simulink model "PMSM"  (R2024b)
settings: Solver=VariableStepAuto  StartTime=0.0  StopTime=1  RelTol=1e-3
InitFcn:
  | Rs=2.98;
  | Ld=7*10^-3;
  | Lq=7*10^-3;
  | pm=0.125;
  | p=2;
  | B=11*10^-5;
  | J=0.47*10^-4;
libraries: spsPLL3phLib x1, spsabctoAlphaBetaZeroLib x1, spsabctodq0Lib x1
settings Model: Creator=krishanchoudhary  LastModifiedBy=krishanchoudhary

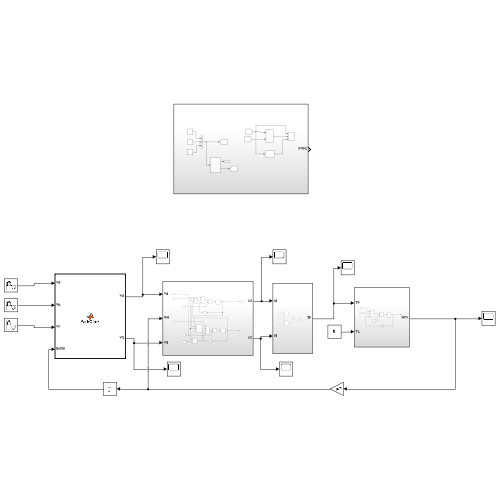
[thumbnail: Simulink's stored preview of the top-level diagram]
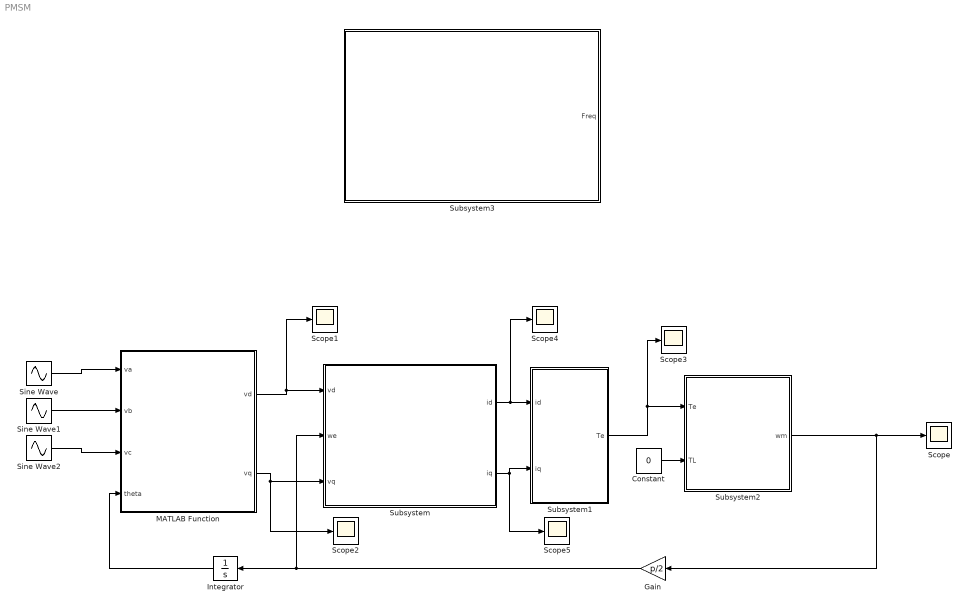
== system PMSM ==
  Constant : Constant  Value=0
  Gain : Gain  Gain=p/2
  Integrator : Integrator
  MATLAB Function : MATLAB Function  TreatAsAtomicUnit=on
  Scope{,1..5} (6 alike) : Scope
  Sine Wave : Sin  Amplitude=240  Frequency=2*pi*50  SampleTime=0.001
  Sine Wave1 : Sin  Amplitude=240  Frequency=2*pi*50  Phase=-(2*pi)/3  SampleTime=0.001
  Sine Wave2 : Sin  Amplitude=240  Frequency=2*pi*50  Phase=(2*pi)/3  SampleTime=0.001
  Subsystem : Subsystem
  Subsystem1 : Subsystem
  Subsystem2 : Subsystem
  Subsystem3 : Subsystem
  wires:
  Subsystem/1(id) -> Scope4/1, Subsystem1/1(id)
  Subsystem/2(iq) -> Scope5/1, Subsystem1/2(iq)
  Subsystem1/1(Te) -> Scope3/1, Subsystem2/1(Te)
  Constant/1 -> Subsystem2/2(TL)
  Subsystem2/1(wm) -> Scope/1, Gain/1
  MATLAB Function/1(vd) -> Scope1/1, Subsystem/1(vd)
  MATLAB Function/2(vq) -> Scope2/1, Subsystem/3(vq)
  Integrator/1 -> MATLAB Function/4(theta)
  Gain/1 -> Subsystem/2(we), Integrator/1
  Sine Wave/1 -> MATLAB Function/1(va)
  Sine Wave1/1 -> MATLAB Function/2(vb)
  Sine Wave2/1 -> MATLAB Function/3(vc)

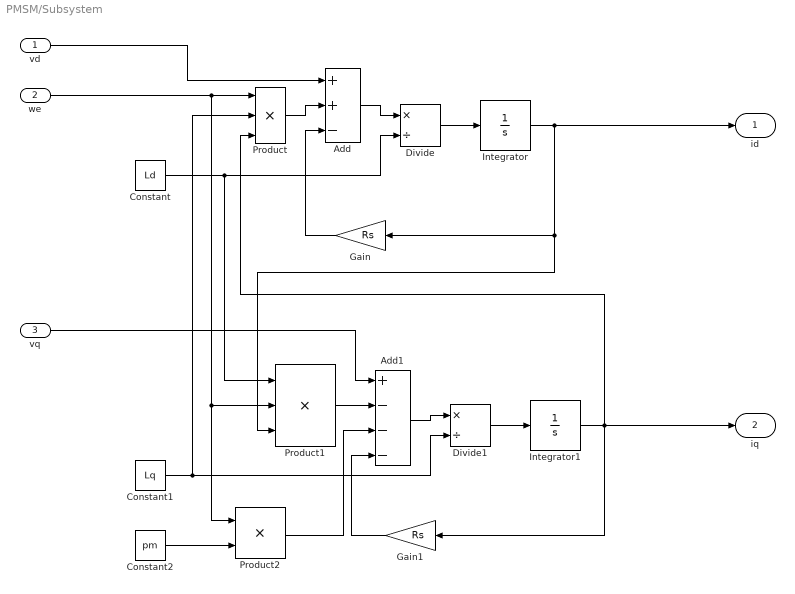
== system PMSM/Subsystem ==
  vd : Inport
  we : Inport  Port=2
  vq : Inport  Port=3
  Add : Sum  Inputs=++-
  Add1 : Sum  Inputs=+---
  Constant : Constant  Value=Ld
  Constant1 : Constant  Value=Lq
  Constant2 : Constant  Value=pm
  Divide : Product  Inputs=*/
  Divide1 : Product  Inputs=*/
  Gain : Gain  Gain=Rs
  Gain1 : Gain  Gain=Rs
  Integrator : Integrator
  Integrator1 : Integrator
  Product : Product  Inputs=3
  Product1 : Product  Inputs=3
  Product2 : Product
  id : Outport
  iq : Outport  Port=2
  wires:
  Constant2/1 -> Product2/2
  Integrator1/1 -> iq/1, Product/3, Gain1/1
  Product2/1 -> Add1/3
  Constant1/1 -> Divide1/2, Product/2
  Product/1 -> Add/2
  Gain1/1 -> Add1/4
  Constant/1 -> Product1/1, Divide/2
  we/1 -> Product/1, Product2/1, Product1/2
  Divide/1 -> Integrator/1
  Gain/1 -> Add/3
  Product1/1 -> Add1/2
  Integrator/1 -> id/1, Gain/1, Product1/3
  vq/1 -> Add1/1
  Divide1/1 -> Integrator1/1
  Add/1 -> Divide/1
  Add1/1 -> Divide1/1
  vd/1 -> Add/1

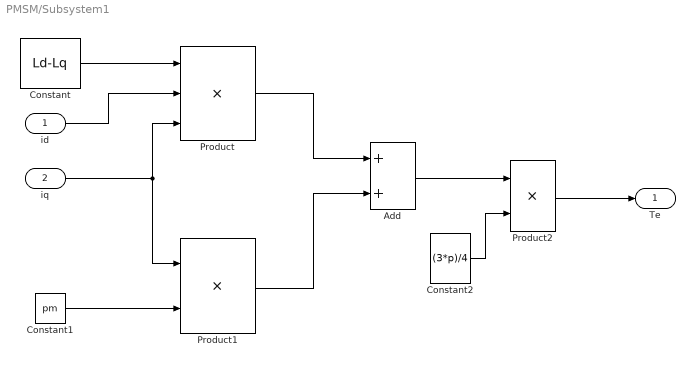
== system PMSM/Subsystem1 ==
  id : Inport
  iq : Inport  Port=2
  Add : Sum
  Constant : Constant  Value=Ld-Lq
  Constant1 : Constant  Value=pm
  Constant2 : Constant  Value=(3*p)/4
  Product : Product  Inputs=3
  Product1 : Product
  Product2 : Product
  Te : Outport
  wires:
  Add/1 -> Product2/1
  Product2/1 -> Te/1
  iq/1 -> Product1/1, Product/3
  id/1 -> Product/2
  Product/1 -> Add/1
  Constant/1 -> Product/1
  Constant2/1 -> Product2/2
  Product1/1 -> Add/2
  Constant1/1 -> Product1/2

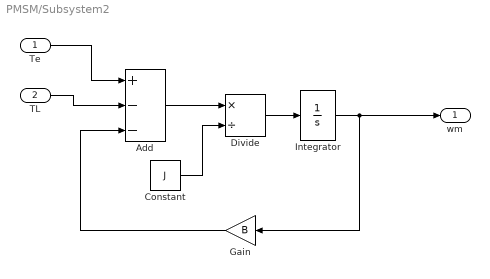
== system PMSM/Subsystem2 ==
  Te : Inport
  TL : Inport  Port=2
  Add : Sum  Inputs=+--
  Constant : Constant  Value=J
  Divide : Product  Inputs=*/
  Gain : Gain  Gain=B
  Integrator : Integrator
  wm : Outport
  wires:
  Add/1 -> Divide/1
  Divide/1 -> Integrator/1
  Gain/1 -> Add/3
  TL/1 -> Add/2
  Integrator/1 -> wm/1, Gain/1
  Constant/1 -> Divide/2
  Te/1 -> Add/1

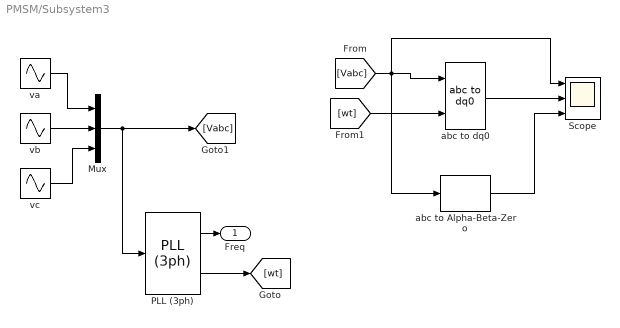
== system PMSM/Subsystem3 ==
  Mux : Mux  Inputs=3
  PLL (3ph) : spsPLL3phLib/PLL (3ph)  Fmin=45  Par_Init=[0, 50]  ParK=[180, 3200, 1]  TcD=1e-4  MaxRateChangeFreq=12  FilterCutOffFreq=25  Ts=0  AGC=on
  Scope : Scope  NumInputPorts=3
      settings: Priority=3
  abc to Alpha-Beta-Zero : spsabctoAlphaBetaZeroLib/abc to Alpha-Beta-Zero
  abc to dq0 : spsabctodq0Lib/abc to dq0  Alignment=90 degrees behind phase A axis
  va : Sin  Amplitude=240  Frequency=2*pi*50  SampleTime=0
  vb : Sin  Amplitude=240  Frequency=2*pi*50  Phase=(-120/360)*2*pi  SampleTime=0
  vc : Sin  Amplitude=240  Frequency=2*pi*50  Phase=(120/360)*2*pi  SampleTime=0
  Freq : Outport
  wires:
  PLL (3ph)/2 -> [wt]
  abc to Alpha-Beta-Zero/1 -> Scope/3
  vc/1 -> Mux/3
  Mux/1 -> [Vabc], PLL (3ph)/1
  PLL (3ph)/1 -> Freq/1
  [wt] -> abc to dq0/2
  abc to dq0/1 -> Scope/2
  vb/1 -> Mux/2
  va/1 -> Mux/1
  [Vabc] -> Scope/1, abc to Alpha-Beta-Zero/1, abc to dq0/1

== matlab function PMSM/MATLAB Function ==
  data: va input; vd output; vb input; vc input; theta input; vq output
function [vd,vq]= ParkClark(va,vb,vc,theta)
if isempty(theta)
theta=o;
end
vd=(2/3)*(va*cos(theta)+vb*cos(theta-(2*pi/3))+vc*cos(theta+(2*pi/3)));
vq=(2/3)*(-va*sin(theta)-vb*sin(theta-(2*pi/3))-vc*sin(theta+(2*pi/3)));
end
